simulink model "Sim_tanksmodel_Astar"  (R2020b)
settings: Solver=FixedStepAuto  StartTime=0.0  StopTime=1500  FixedStep=1  RelTol=1e-3  EnableMultiTasking=on
InitFcn:
  | cd ..
  | addpath(genpath('Algoritmo'))
  | cd ..
  | addpath(genpath('Sistema-Multitanque'))
  | cd AS-PID\Simulacion
  | inParameters
StopFcn:
  | BestGains1 = [AS(1).Kp AS(1).Ki AS(1).Kd];
  | BestGains2 = [AS(2).Kp AS(2).Ki AS(2).Kd];
  | BestGains3 = [AS(3).Kp AS(3).Ki AS(3).Kd];
  | save('deletetoreset.mat','BestGains1','BestGains2','BestGains3')
values from neighbouring files (symbols this model uses):
  Ts = AS_vars(2)    [sfun_Astar.m]
undefined symbols (not defined in the file or in its folder): AS, he1, he2, Kd1, Kd2, Kd3, Ki1, Ki2, Ki3, Kp1, Kp2, Kp3
libraries: simulink x2
settings Model: SimulationMode=accelerator  Creator=sahandar  LastModifiedBy=Usuario
settings SolverCC: AlgebraicLoopSolver=LineSearch  AutoInsertRateTranBlk=on
settings DataIOCC: LimitDataPoints=on  SaveFormat=Array  ReturnWorkspaceOutputs=off
settings OptimizationCC: LifeSpan=inf
settings DebuggingCC: AllowSymbolicDim=off  SFUnexpectedBacktrackingDiag=warning  SFNoUnconditionalDefaultTransitionDiag=warning  SFExecutionAtInitializationDiag=none  ArithmeticOperatorsInVariantConditions=warning
settings HardwareCC: ProdBitPerPointer=32  ProdBitPerSizeT=32  ProdBitPerPtrDiffT=32  ProdLargestAtomicFloat=None  ProdIntDivRoundTo=Undefined  ProdEndianess=Unspecified  ProdWordSize=32  ProdHWDeviceType=32-bit Generic
settings ModelReferenceCC: PropagateSignalLabelsOutOfModel=off
settings SFSimCC: SimUseLocalCustomCode=off  CustomCodeUndefinedFunction=UseInterfaceOnly
settings RTWCC: RTWUseLocalCustomCode=off
settings CodeAppCC: StateflowObjectComments=on
settings GRTTargetCC: TargetLangStandard=C89/C90 (ANSI)
settings ConfigComp: CovMetricSettings=dw  CovSaveCumulativeToWorkspaceVar=on  CovSaveSingleToWorkspaceVar=on  CovExternalEMLEnable=off

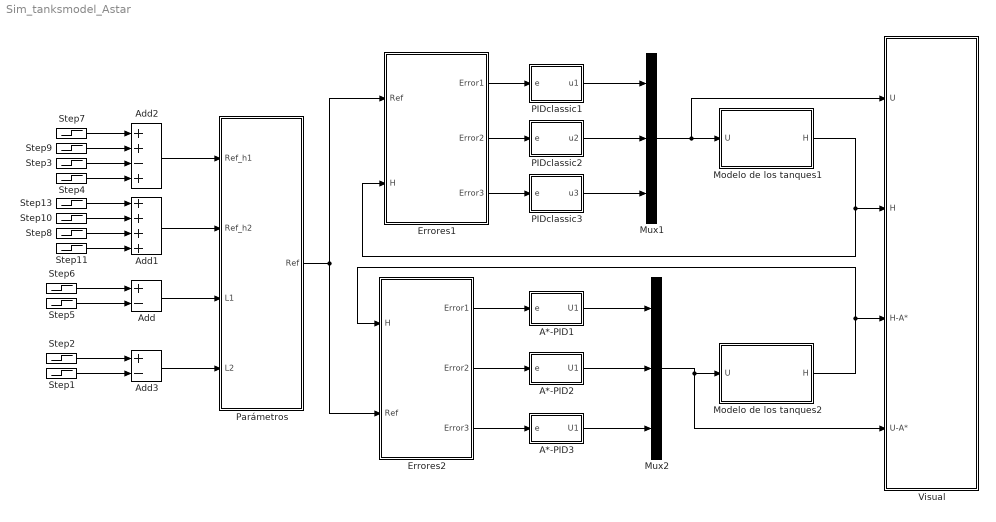
== system Sim_tanksmodel_Astar ==
  A*-PID1 : Subsystem
  A*-PID2 : Subsystem
  A*-PID3 : Subsystem
  Add : Sum  Inputs=+-
  Add1 : Sum  Inputs=++++
  Add2 : Sum  Inputs=++-+
  Add3 : Sum  Inputs=+-
  Errores1 : Subsystem
  Errores2 : Subsystem
  Modelo de los tanques1 : Subsystem
  Modelo de los tanques2 : Subsystem
  Mux1 : Mux  Inputs=3
  Mux2 : Mux  Inputs=3
  PIDclassic1 : Subsystem
  PIDclassic2 : Subsystem
  PIDclassic3 : Subsystem
  Parámetros : Subsystem
  Step1 : Step  Time=900  SampleTime=Ts
  Step10 : Step  Time=350  After=-0.03  SampleTime=Ts
  Step11 : Step  Time=1100  After=-0.03  SampleTime=Ts
  Step13 : Step  Time=0  Before=he2  After=0.05  SampleTime=Ts
  Step2 : Step  Time=800  SampleTime=Ts
  Step3 : Step  Time=700  After=0.05  SampleTime=Ts
  Step4 : Step  Time=1100  After=0.05  SampleTime=Ts
  Step5 : Step  Time=800  SampleTime=Ts
  Step6 : Step  Time=600  SampleTime=Ts
  Step7 : Step  Time=0  Before=he1  After=0.15  SampleTime=Ts
  Step8 : Step  Time=700  After=0.02  SampleTime=Ts
  Step9 : Step  Time=350  After=0.05  SampleTime=Ts
  Visual : Subsystem
  wires:
  Mux1/1 -> Visual/1(U), Modelo de los tanques1/1(U)
  Step6/1 -> Add/1
  Step5/1 -> Add/2
  Modelo de los tanques1/1(H) -> Errores1/2(H), Visual/2(H)
  Step1/1 -> Add3/2
  Step2/1 -> Add3/1
  Errores2/1(Error1) -> A*-PID1/1(e)
  Modelo de los tanques2/1(H) -> Visual/3(H-A*), Errores2/1(H)
  Parámetros/1(Ref) -> Errores2/2(Ref), Errores1/1(Ref)
  Mux2/1 -> Visual/4(U-A*), Modelo de los tanques2/1(U)
  PIDclassic2/1(u2) -> Mux1/2
  PIDclassic3/1(u3) -> Mux1/3
  Errores1/2(Error2) -> PIDclassic2/1(e)
  Errores1/3(Error3) -> PIDclassic3/1(e)
  Errores1/1(Error1) -> PIDclassic1/1(e)
  PIDclassic1/1(u1) -> Mux1/1
  Add2/1 -> Parámetros/1(Ref_h1)
  Add1/1 -> Parámetros/2(Ref_h2)
  A*-PID1/1(U1) -> Mux2/1
  Step7/1 -> Add2/1
  Step13/1 -> Add1/1
  Step10/1 -> Add1/2
  Step9/1 -> Add2/2
  Step3/1 -> Add2/3
  Step4/1 -> Add2/4
  Errores2/2(Error2) -> A*-PID2/1(e)
  A*-PID2/1(U1) -> Mux2/2
  Errores2/3(Error3) -> A*-PID3/1(e)
  A*-PID3/1(U1) -> Mux2/3
  Step8/1 -> Add1/3
  Step11/1 -> Add1/4
  Add/1 -> Parámetros/3(L1)
  Add3/1 -> Parámetros/4(L2)

== system Sim_tanksmodel_Astar/A*-PID1 ==
  e : Inport
  Demux : Demux  Outputs=3
  Mux : Mux
  PID Controller : Subsystem
  S-Function : S-Function  FunctionName=sfun_Astar  Parameters=AS_vars1  SFunctionDeploymentMode=off  EnableBusSupport=off
  Saturation1 : Saturate  UpperLimit=1  LowerLimit=0
  Scope : Scope  NumInputPorts=3
  Subsystem : Subsystem
  U1 : Outport
  wires:
  Saturation1/1 -> U1/1
  PID Controller/1(u) -> Saturation1/1
  Mux/1 -> S-Function/1
  Subsystem/1(ref) -> Mux/2
  Subsystem/2(enable) -> Mux/3
  S-Function/1 -> Demux/1
  Demux/3 -> Scope/3, PID Controller/4(Kd)  "Kd"
  e/1 -> Mux/1, PID Controller/1(e)
  Subsystem/3(iter) -> Mux/4
  Demux/1 -> Scope/1, PID Controller/2(Kp)  "Kp"
  Demux/2 -> Scope/2, PID Controller/3(Ki)  "Ki"

== system Sim_tanksmodel_Astar/A*-PID2 ==
  e : Inport
  Demux : Demux  Outputs=3
  Mux : Mux
  PID Controller : Subsystem
  S-Function : S-Function  FunctionName=sfun_Astar  Parameters=AS_vars2  SFunctionDeploymentMode=off  EnableBusSupport=off
  Saturation1 : Saturate  UpperLimit=1  LowerLimit=0
  Scope : Scope  NumInputPorts=3
  Subsystem : Subsystem
  U1 : Outport
  wires:
  Demux/2 -> PID Controller/3(Ki), Scope/2  "Ki"
  Demux/1 -> PID Controller/2(Kp), Scope/1  "Kp"
  Subsystem/3(iter) -> Mux/4
  e/1 -> PID Controller/1(e), Mux/1
  Demux/3 -> PID Controller/4(Kd), Scope/3  "Kd"
  S-Function/1 -> Demux/1
  Subsystem/2(enable) -> Mux/3
  Subsystem/1(ref) -> Mux/2
  Mux/1 -> S-Function/1
  Saturation1/1 -> U1/1
  PID Controller/1(u) -> Saturation1/1

== system Sim_tanksmodel_Astar/A*-PID3 ==
  e : Inport
  Demux : Demux  Outputs=3
  Gain : Gain  Gain=-1
  Mux : Mux
  PID Controller : Subsystem
  S-Function : S-Function  FunctionName=sfun_Astar  Parameters=AS_vars3  SFunctionDeploymentMode=off  EnableBusSupport=off
  Saturation1 : Saturate  UpperLimit=1  LowerLimit=0
  Scope : Scope  NumInputPorts=3
  Subsystem : Subsystem
  U1 : Outport
  wires:
  Saturation1/1 -> U1/1
  Mux/1 -> S-Function/1
  Subsystem/1(ref) -> Mux/2
  Subsystem/2(enable) -> Mux/3
  S-Function/1 -> Demux/1
  Demux/3 -> Scope/3, PID Controller/4(Kd)  "Kd"
  e/1 -> Mux/1, PID Controller/1(e)
  Subsystem/3(iter) -> Mux/4
  Demux/1 -> Scope/1, PID Controller/2(Kp)  "Kp"
  Demux/2 -> Scope/2, PID Controller/3(Ki)  "Ki"
  PID Controller/1(u) -> Gain/1
  Gain/1 -> Saturation1/1

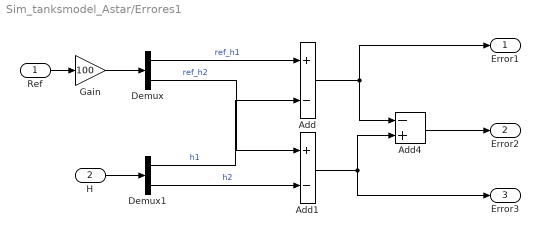
== system Sim_tanksmodel_Astar/Errores1 ==
  Ref : Inport
  H : Inport  Port=2
  Add : Sum  Inputs=+-
  Add1 : Sum  Inputs=+-
  Add4 : Sum  Inputs=-+
  Demux : Demux  Outputs=2
  Demux1 : Demux  Outputs=2
  Gain : Gain  Gain=100
  Error1 : Outport
  Error2 : Outport  Port=2
  Error3 : Outport  Port=3
  wires:
  Add4/1 -> Error2/1
  H/1 -> Demux1/1
  Demux/1 -> Add/1  "ref_h1"
  Demux1/1 -> Add/2  "h1"
  Ref/1 -> Gain/1
  Add/1 -> Add4/1, Error1/1
  Demux1/2 -> Add1/2  "h2"
  Add1/1 -> Add4/2, Error3/1
  Demux/2 -> Add1/1  "ref_h2"
  Gain/1 -> Demux/1

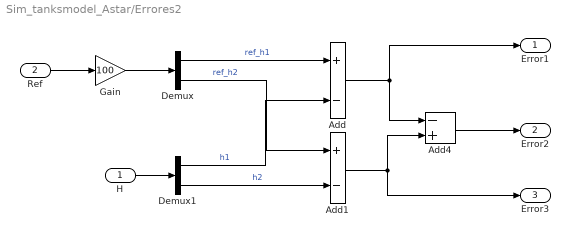
== system Sim_tanksmodel_Astar/Errores2 ==
  H : Inport
  Ref : Inport  Port=2
  Add : Sum  Inputs=+-
  Add1 : Sum  Inputs=+-
  Add4 : Sum  Inputs=-+
  Demux : Demux  Outputs=2
  Demux1 : Demux  Outputs=2
  Gain : Gain  Gain=100
  Error1 : Outport
  Error2 : Outport  Port=2
  Error3 : Outport  Port=3
  wires:
  Add4/1 -> Error2/1
  H/1 -> Demux1/1
  Demux/1 -> Add/1  "ref_h1"
  Demux1/1 -> Add/2  "h1"
  Ref/1 -> Gain/1
  Add/1 -> Add4/1, Error1/1
  Demux1/2 -> Add1/2  "h2"
  Add1/1 -> Add4/2, Error3/1
  Demux/2 -> Add1/1  "ref_h2"
  Gain/1 -> Demux/1

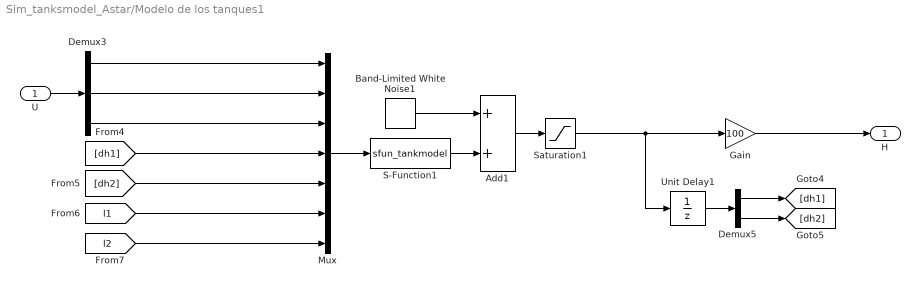
== system Sim_tanksmodel_Astar/Modelo de los tanques1 ==
  U : Inport
  Add1 : Sum
  Band-Limited White Noise1 : simulink/Sources/Band-Limited White Noise  Cov=N  Ts=Ts  seed=[23341]
  Demux3 : Demux  Outputs=3
  Demux5 : Demux  Outputs=2
  Gain : Gain  Gain=100
  Mux : Mux  Inputs=7
  S-Function1 : S-Function  FunctionName=sfun_tankmodel  Parameters=vars  SFunctionDeploymentMode=off  EnableBusSupport=off
  Saturation1 : Saturate  UpperLimit=0.25  LowerLimit=0
  Unit Delay1 : UnitDelay  SampleTime=-1  HasFrameUpgradeWarning=on
  H : Outport  VectorParamsAs1DForOutWhenUnconnected=off
  wires:
  Saturation1/1 -> Unit Delay1/1, Gain/1
  Demux3/2 -> Mux/2
  Band-Limited White Noise1/1 -> Add1/1
  [l2] -> Mux/7
  [l1] -> Mux/6
  S-Function1/1 -> Add1/2
  [dh2] -> Mux/5
  Demux3/3 -> Mux/3
  Add1/1 -> Saturation1/1
  U/1 -> Demux3/1
  Demux3/1 -> Mux/1
  [dh1] -> Mux/4
  Mux/1 -> S-Function1/1
  Unit Delay1/1 -> Demux5/1
  Demux5/1 -> [dh1]
  Demux5/2 -> [dh2]
  Gain/1 -> H/1

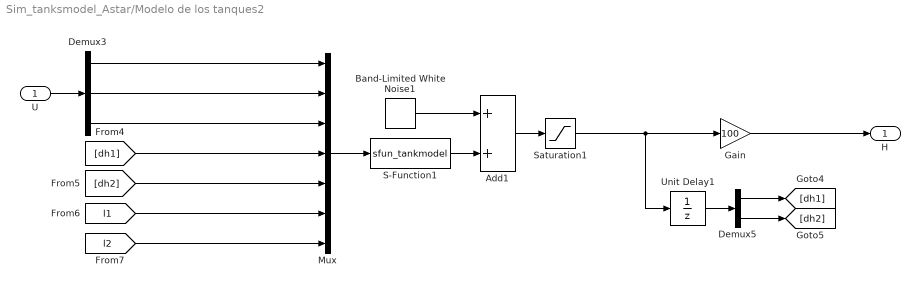
== system Sim_tanksmodel_Astar/Modelo de los tanques2 ==
  U : Inport
  Add1 : Sum
  Band-Limited White Noise1 : simulink/Sources/Band-Limited White Noise  Cov=N  Ts=Ts  seed=[23341]
  Demux3 : Demux  Outputs=3
  Demux5 : Demux  Outputs=2
  Gain : Gain  Gain=100
  Mux : Mux  Inputs=7
  S-Function1 : S-Function  FunctionName=sfun_tankmodel  Parameters=vars  SFunctionDeploymentMode=off  EnableBusSupport=off
  Saturation1 : Saturate  UpperLimit=0.25  LowerLimit=0
  Unit Delay1 : UnitDelay  SampleTime=-1  HasFrameUpgradeWarning=on
  H : Outport  VectorParamsAs1DForOutWhenUnconnected=off
  wires:
  Demux5/2 -> [dh2]
  Demux5/1 -> [dh1]
  Unit Delay1/1 -> Demux5/1
  Mux/1 -> S-Function1/1
  [dh1] -> Mux/4
  Demux3/1 -> Mux/1
  U/1 -> Demux3/1
  Add1/1 -> Saturation1/1
  Demux3/3 -> Mux/3
  [dh2] -> Mux/5
  S-Function1/1 -> Add1/2
  [l1] -> Mux/6
  [l2] -> Mux/7
  Band-Limited White Noise1/1 -> Add1/1
  Demux3/2 -> Mux/2
  Saturation1/1 -> Gain/1, Unit Delay1/1
  Gain/1 -> H/1

== system Sim_tanksmodel_Astar/PIDclassic1 ==
  e : Inport
  Constant : Constant  Value=Kp1
  Constant1 : Constant  Value=Ki1
  Constant2 : Constant  Value=Kd1
  PID Controller : Subsystem
  Saturation : Saturate  UpperLimit=1  LowerLimit=0
  u1 : Outport
  wires:
  Constant2/1 -> PID Controller/4(Kd)
  Constant1/1 -> PID Controller/3(Ki)
  Constant/1 -> PID Controller/2(Kp)
  e/1 -> PID Controller/1(e)
  PID Controller/1(u) -> Saturation/1
  Saturation/1 -> u1/1

== system Sim_tanksmodel_Astar/PIDclassic2 ==
  e : Inport
  Constant : Constant  Value=Kp2
  Constant1 : Constant  Value=Ki2
  Constant2 : Constant  Value=Kd2
  PID Controller : Subsystem
  Saturation : Saturate  UpperLimit=1  LowerLimit=0
  u2 : Outport
  wires:
  Saturation/1 -> u2/1
  e/1 -> PID Controller/1(e)
  Constant/1 -> PID Controller/2(Kp)
  Constant1/1 -> PID Controller/3(Ki)
  Constant2/1 -> PID Controller/4(Kd)
  PID Controller/1(u) -> Saturation/1

== system Sim_tanksmodel_Astar/PIDclassic3 ==
  e : Inport
  Constant : Constant  Value=Kp3
  Constant1 : Constant  Value=Ki3
  Constant2 : Constant  Value=Kd3
  Gain : Gain  Gain=-1
  PID Controller : Subsystem
  Saturation : Saturate  UpperLimit=1  LowerLimit=0
  u3 : Outport
  wires:
  Constant2/1 -> PID Controller/4(Kd)
  Constant1/1 -> PID Controller/3(Ki)
  Constant/1 -> PID Controller/2(Kp)
  e/1 -> PID Controller/1(e)
  Saturation/1 -> u3/1
  PID Controller/1(u) -> Gain/1
  Gain/1 -> Saturation/1

== system Sim_tanksmodel_Astar/Parámetros ==
  Ref_h1 : Inport
  Ref_h2 : Inport  Port=2
  L1 : Inport  Port=3
  L2 : Inport  Port=4
  Mux : Mux  Inputs=2
  Ref : Outport
  tag scope: l1=global, l2=global, ref_h1=global, ref_h2=global
  wires:
  L1/1 -> [l1]
  Mux/1 -> Ref/1
  Ref_h1/1 -> [ref_h1], Mux/1
  L2/1 -> [l2]
  Ref_h2/1 -> Mux/2, [ref_h2]

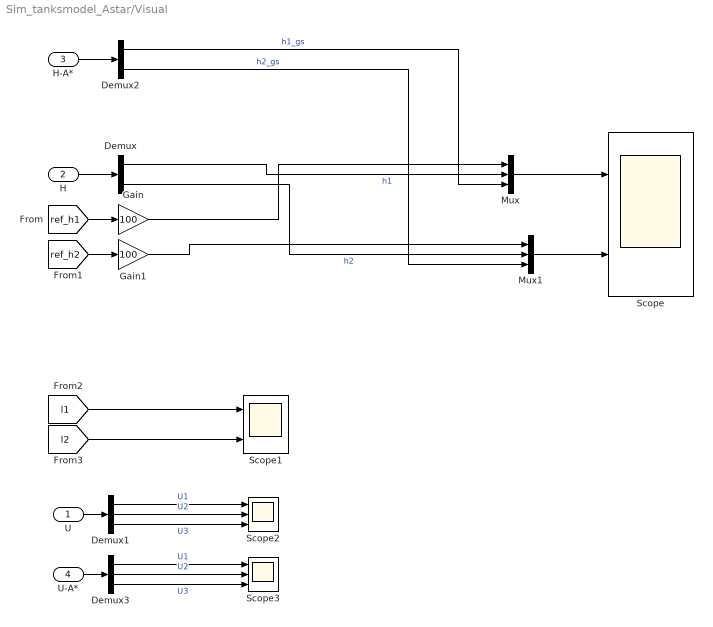
== system Sim_tanksmodel_Astar/Visual ==
  U : Inport
  H : Inport  Port=2
  H-A* : Inport  Port=3
  U-A* : Inport  Port=4
  Demux : Demux  Outputs=2
  Demux1 : Demux  Outputs=3
  Demux2 : Demux  Outputs=2
  Demux3 : Demux  Outputs=3
  Gain : Gain  Gain=100
  Gain1 : Gain  Gain=100
  Mux : Mux  Inputs=3
  Mux1 : Mux  Inputs=3
  Scope : Scope  NumInputPorts=2
  Scope1 : Scope  NumInputPorts=2
  Scope2 : Scope  NumInputPorts=3
  Scope3 : Scope  NumInputPorts=3
  wires:
  H/1 -> Demux/1
  Demux/1 -> Mux/2  "h1"
  [ref_h1] -> Gain/1
  Mux/1 -> Scope/1
  Demux/2 -> Mux1/2  "h2"
  [ref_h2] -> Gain1/1
  [l1] -> Scope1/1
  [l2] -> Scope1/2
  U/1 -> Demux1/1
  Demux1/1 -> Scope2/1  "U1"
  Demux1/2 -> Scope2/2  "U2"
  Demux1/3 -> Scope2/3  "U3"
  Mux1/1 -> Scope/2
  Demux2/1 -> Mux/3  "h1_gs"
  H-A*/1 -> Demux2/1
  Demux2/2 -> Mux1/3  "h2_gs"
  Demux3/2 -> Scope3/2  "U2"
  Demux3/1 -> Scope3/1  "U1"
  U-A*/1 -> Demux3/1
  Demux3/3 -> Scope3/3  "U3"
  Gain/1 -> Mux/1
  Gain1/1 -> Mux1/1

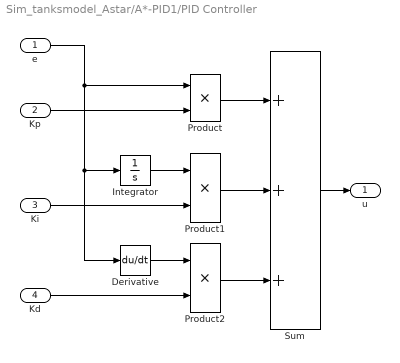
== system Sim_tanksmodel_Astar/A*-PID1/PID Controller ==
  e : Inport
  Kp : Inport  Port=2
  Ki : Inport  Port=3
  Kd : Inport  Port=4
  Derivative : Derivative
  Integrator : Integrator
  Product : Product
  Product1 : Product
  Product2 : Product
  Sum : Sum  Inputs=3
  u : Outport
  wires:
  Sum/1 -> u/1
  Product/1 -> Sum/1
  Kp/1 -> Product/2
  Ki/1 -> Product1/2
  Integrator/1 -> Product1/1
  Product1/1 -> Sum/2
  Product2/1 -> Sum/3
  Kd/1 -> Product2/2
  e/1 -> Derivative/1, Integrator/1, Product/1
  Derivative/1 -> Product2/1

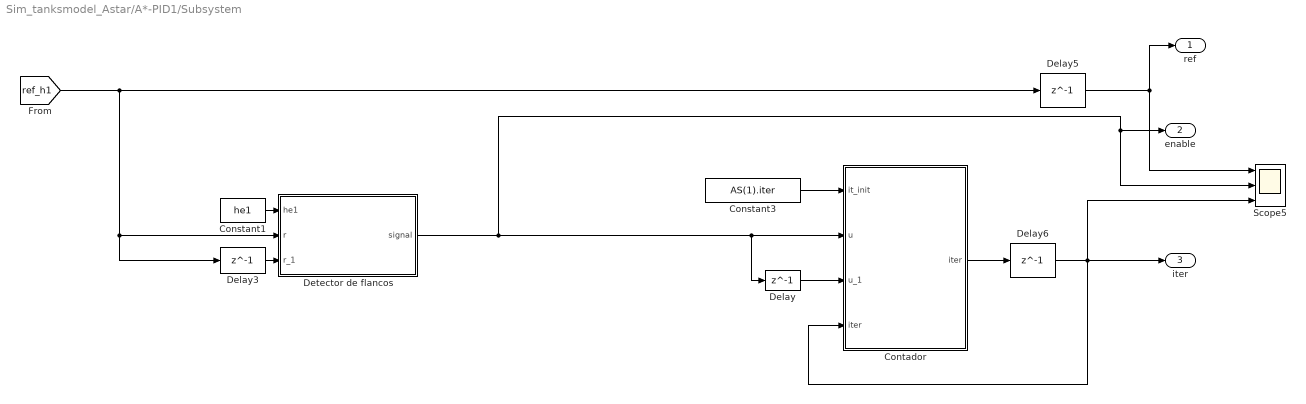
== system Sim_tanksmodel_Astar/A*-PID1/Subsystem ==
  Constant1 : Constant  Value=he1
  Constant3 : Constant  Value=AS(1).iter
  Contador : MATLAB Function  TreatAsAtomicUnit=on
  Delay : Delay  DelayLength=1  InitialCondition=0
  Delay3 : Delay  DelayLength=1  InitialCondition=he1
  Delay5 : Delay  DelayLength=1  InitialCondition=0
  Delay6 : Delay  DelayLength=1  InitialCondition=0
  Detector de flancos : MATLAB Function  TreatAsAtomicUnit=on
  Scope5 : Scope  NumInputPorts=3
  ref : Outport
  enable : Outport  Port=2
  iter : Outport  Port=3
  wires:
  Contador/1(iter) -> Delay6/1
  Delay/1 -> Contador/3(u_1)
  [ref_h1] -> Delay3/1, Detector de flancos/2(r), Delay5/1
  Delay3/1 -> Detector de flancos/3(r_1)
  Delay5/1 -> Scope5/1, ref/1
  Delay6/1 -> Scope5/3, iter/1, Contador/4("iter ")
  Detector de flancos/1(signal) -> Delay/1, Contador/2(u), Scope5/2, enable/1
  Constant1/1 -> Detector de flancos/1(he1)
  Constant3/1 -> Contador/1(it_init)

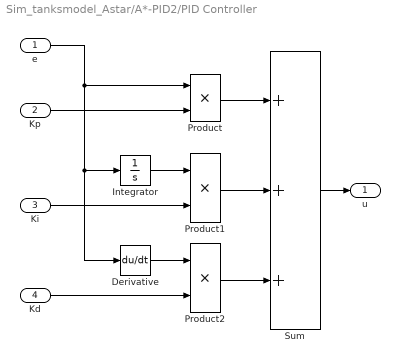
== system Sim_tanksmodel_Astar/A*-PID2/PID Controller ==
  e : Inport
  Kp : Inport  Port=2
  Ki : Inport  Port=3
  Kd : Inport  Port=4
  Derivative : Derivative
  Integrator : Integrator
  Product : Product
  Product1 : Product
  Product2 : Product
  Sum : Sum  Inputs=3
  u : Outport
  wires:
  Derivative/1 -> Product2/1
  e/1 -> Product/1, Integrator/1, Derivative/1
  Kd/1 -> Product2/2
  Product2/1 -> Sum/3
  Product1/1 -> Sum/2
  Integrator/1 -> Product1/1
  Ki/1 -> Product1/2
  Kp/1 -> Product/2
  Product/1 -> Sum/1
  Sum/1 -> u/1

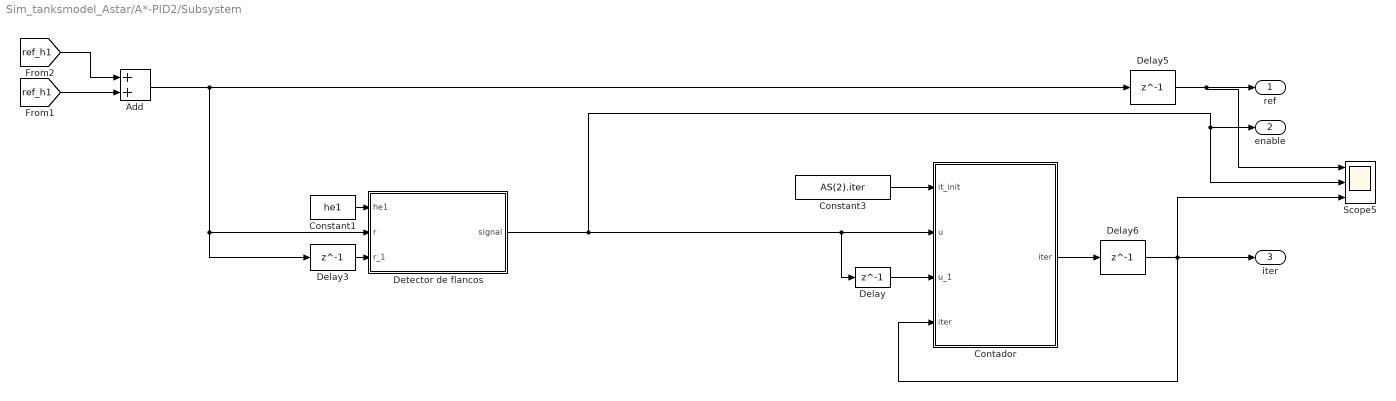
== system Sim_tanksmodel_Astar/A*-PID2/Subsystem ==
  Add : Sum
  Constant1 : Constant  Value=he1
  Constant3 : Constant  Value=AS(2).iter
  Contador : MATLAB Function  TreatAsAtomicUnit=on
  Delay : Delay  DelayLength=1  InitialCondition=0
  Delay3 : Delay  DelayLength=1  InitialCondition=he1
  Delay5 : Delay  DelayLength=1  InitialCondition=0
  Delay6 : Delay  DelayLength=1  InitialCondition=0
  Detector de flancos : MATLAB Function  TreatAsAtomicUnit=on
  Scope5 : Scope  NumInputPorts=3
  ref : Outport
  enable : Outport  Port=2
  iter : Outport  Port=3
  wires:
  Constant3/1 -> Contador/1(it_init)
  Constant1/1 -> Detector de flancos/1(he1)
  Detector de flancos/1(signal) -> enable/1, Scope5/2, Contador/2(u), Delay/1
  Delay6/1 -> Contador/4("iter "), iter/1, Scope5/3
  Delay5/1 -> ref/1, Scope5/1
  Delay3/1 -> Detector de flancos/3(r_1)
  Add/1 -> Delay5/1, Detector de flancos/2(r), Delay3/1
  Delay/1 -> Contador/3(u_1)
  Contador/1(iter) -> Delay6/1
  [ref_h1] -> Add/2
  [ref_h1] -> Add/1

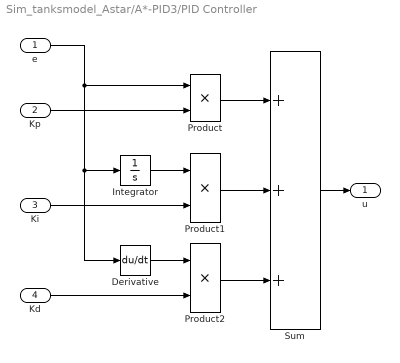
== system Sim_tanksmodel_Astar/A*-PID3/PID Controller ==
  e : Inport
  Kp : Inport  Port=2
  Ki : Inport  Port=3
  Kd : Inport  Port=4
  Derivative : Derivative
  Integrator : Integrator
  Product : Product
  Product1 : Product
  Product2 : Product
  Sum : Sum  Inputs=3
  u : Outport
  wires:
  Sum/1 -> u/1
  Product/1 -> Sum/1
  Kp/1 -> Product/2
  Ki/1 -> Product1/2
  Integrator/1 -> Product1/1
  Product1/1 -> Sum/2
  Product2/1 -> Sum/3
  Kd/1 -> Product2/2
  e/1 -> Derivative/1, Integrator/1, Product/1
  Derivative/1 -> Product2/1

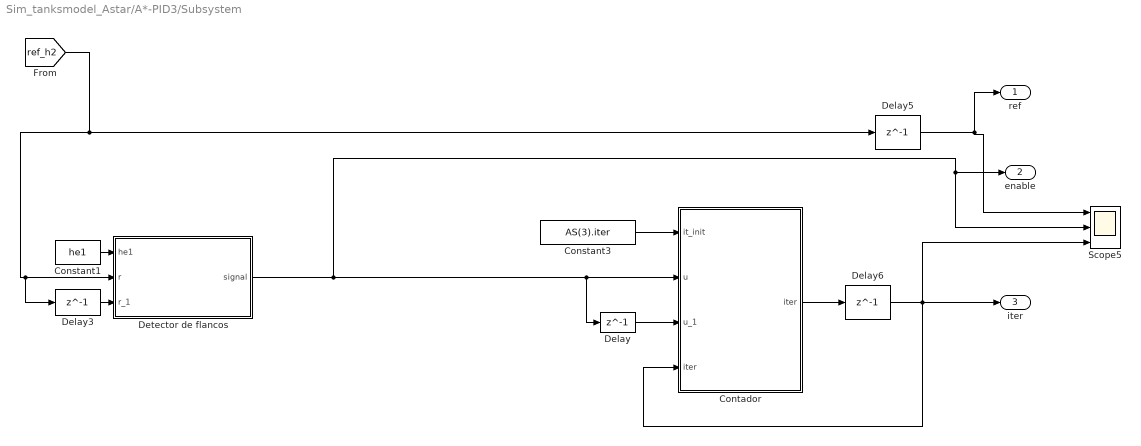
== system Sim_tanksmodel_Astar/A*-PID3/Subsystem ==
  Constant1 : Constant  Value=he1
  Constant3 : Constant  Value=AS(3).iter
  Contador : MATLAB Function  TreatAsAtomicUnit=on
  Delay : Delay  DelayLength=1  InitialCondition=0
  Delay3 : Delay  DelayLength=1  InitialCondition=he1
  Delay5 : Delay  DelayLength=1  InitialCondition=0
  Delay6 : Delay  DelayLength=1  InitialCondition=0
  Detector de flancos : MATLAB Function  TreatAsAtomicUnit=on
  Scope5 : Scope  NumInputPorts=3
  ref : Outport
  enable : Outport  Port=2
  iter : Outport  Port=3
  wires:
  Contador/1(iter) -> Delay6/1
  Delay/1 -> Contador/3(u_1)
  Delay3/1 -> Detector de flancos/3(r_1)
  Delay5/1 -> Scope5/1, ref/1
  Delay6/1 -> Scope5/3, iter/1, Contador/4("iter ")
  Detector de flancos/1(signal) -> Delay/1, Contador/2(u), Scope5/2, enable/1
  Constant1/1 -> Detector de flancos/1(he1)
  Constant3/1 -> Contador/1(it_init)
  [ref_h2] -> Detector de flancos/2(r), Delay3/1, Delay5/1

== system Sim_tanksmodel_Astar/PIDclassic1/PID Controller ==
  e : Inport
  Kp : Inport  Port=2
  Ki : Inport  Port=3
  Kd : Inport  Port=4
  Derivative : Derivative
  Integrator : Integrator
  Product : Product
  Product1 : Product
  Product2 : Product
  Sum : Sum  Inputs=3
  u : Outport
  wires:
  Sum/1 -> u/1
  Product/1 -> Sum/1
  Kp/1 -> Product/2
  Ki/1 -> Product1/2
  Integrator/1 -> Product1/1
  Product1/1 -> Sum/2
  Product2/1 -> Sum/3
  Kd/1 -> Product2/2
  e/1 -> Derivative/1, Integrator/1, Product/1
  Derivative/1 -> Product2/1

== system Sim_tanksmodel_Astar/PIDclassic2/PID Controller ==
  e : Inport
  Kp : Inport  Port=2
  Ki : Inport  Port=3
  Kd : Inport  Port=4
  Derivative : Derivative
  Integrator : Integrator
  Product : Product
  Product1 : Product
  Product2 : Product
  Sum : Sum  Inputs=3
  u : Outport
  wires:
  Derivative/1 -> Product2/1
  e/1 -> Product/1, Integrator/1, Derivative/1
  Kd/1 -> Product2/2
  Product2/1 -> Sum/3
  Product1/1 -> Sum/2
  Integrator/1 -> Product1/1
  Ki/1 -> Product1/2
  Kp/1 -> Product/2
  Product/1 -> Sum/1
  Sum/1 -> u/1

== system Sim_tanksmodel_Astar/PIDclassic3/PID Controller ==
  e : Inport
  Kp : Inport  Port=2
  Ki : Inport  Port=3
  Kd : Inport  Port=4
  Derivative : Derivative
  Integrator : Integrator
  Product : Product
  Product1 : Product
  Product2 : Product
  Sum : Sum  Inputs=3
  u : Outport
  wires:
  Sum/1 -> u/1
  Product/1 -> Sum/1
  Kp/1 -> Product/2
  Ki/1 -> Product1/2
  Integrator/1 -> Product1/1
  Product1/1 -> Sum/2
  Product2/1 -> Sum/3
  Kd/1 -> Product2/2
  e/1 -> Derivative/1, Integrator/1, Product/1
  Derivative/1 -> Product2/1

== matlab function Sim_tanksmodel_Astar/A*-PID1/Subsystem/Detector de flancos ==
  data: he1 input; r input; signal output; r_1 input
function signal = fcn(he1, r,r_1)
y = 0;
if (r~=r_1) && r_1 ~=he1
    y = 1;
end
signal = y;

== matlab function Sim_tanksmodel_Astar/A*-PID1/Subsystem/Contador ==
  data: it_init input; u input; u_1 input; iter output; iter input
function iter  = fcn(it_init, u,u_1,iter)
if iter == 0
    iter = it_init;
end
if u>u_1
    iter =  iter + 1 ;
end

== matlab function Sim_tanksmodel_Astar/A*-PID2/Subsystem/Contador ==
  data: it_init input; u input; u_1 input; iter output; iter input
function iter  = fcn(it_init, u,u_1,iter)
if iter == 0
    iter = it_init;
end
if u>u_1
    iter =  iter + 1 ;
end

== matlab function Sim_tanksmodel_Astar/A*-PID2/Subsystem/Detector de flancos ==
  data: he1 input; r input; signal output; r_1 input
function signal = fcn(he1, r,r_1)
y = 0;
if (r~=r_1) && r_1 ~=he1
    y = 1;
end
signal = y;

== matlab function Sim_tanksmodel_Astar/A*-PID3/Subsystem/Contador ==
  data: it_init input; u input; u_1 input; iter output; iter input
function iter  = fcn(it_init, u,u_1,iter)
if iter == 0
    iter = it_init;
end
if u>u_1
    iter =  iter + 1 ;
end

== matlab function Sim_tanksmodel_Astar/A*-PID3/Subsystem/Detector de flancos ==
  data: he1 input; r input; signal output; r_1 input
function signal = fcn(he1, r,r_1)
y = 0;
if (r~=r_1) && r_1 ~=he1
    y = 1;
end
signal = y;
